simulink model "v2_unittest"  (R2022a)
settings: Solver=VariableStepAuto  StartTime=0.0  StopTime=10.0  RelTol=1e-3
undefined symbols (not defined in the file): sigbuilder_block
libraries: simulink x2
settings Model: Creator=AAMIR  LastModifiedBy=AAMIR

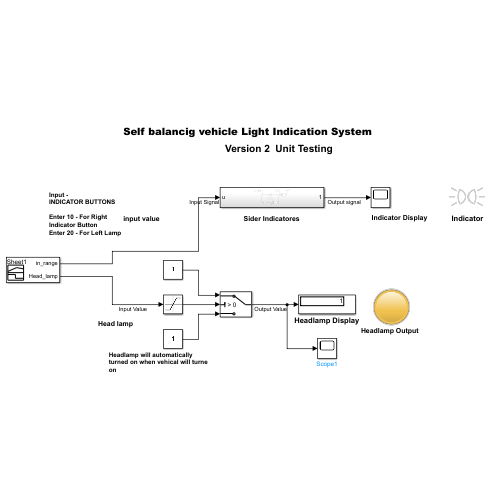
[thumbnail: Simulink's stored preview of the top-level diagram]
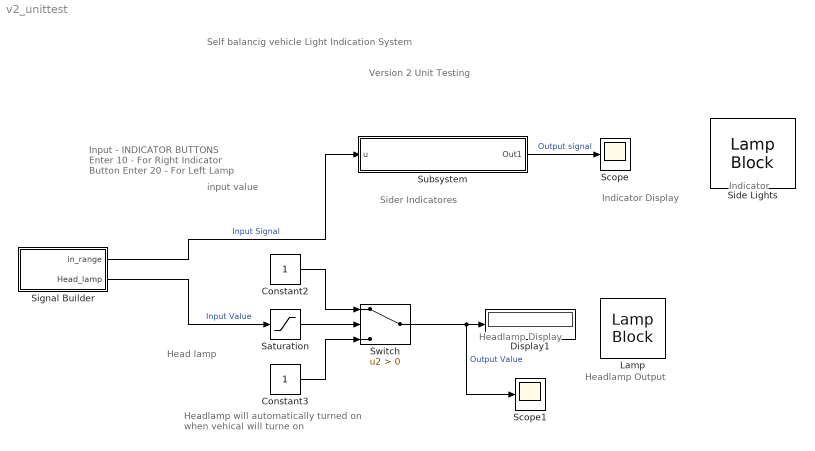
== system v2_unittest ==
  note: input value
  note: Input -
      | INDICATOR BUTTONS
      |
      | Enter 10 - For Right Indicator Button
      | Enter 20 - For Left Lamp
  note: Indicator Display
  note: Head lamp
  note: Self balancig vehicle Light Indication System
  note: Headlamp Output
  note: Indicator
  note: Headlamp will automatically turned on when vehical will turne on
  note: Headlamp Display
  note: Sider Indicatores
  note: Version 2 Unit Testing
  Constant2 : Constant
  Constant3 : Constant
  Display1 : Display
  Lamp : LampBlock  LabelPosition=Hide
  Saturation : Saturate  UpperLimit=1  LowerLimit=0
  Scope : Scope
  Scope1 : Scope
  Side Lights : LampBlock  LabelPosition=Hide  Icon=SideLights
  Signal Builder : Subsystem  Tag=STV Subsys  LoadFcn=sigbuilder_block('load',[437.6 199.2 550.4 400 ]);  StartFcn=sigbuilder_block('start');  StopFcn=sigbuilder_block('stop');  ClipboardFcn=sigbuilder_block('clipboard');  mask(Sigbuilder block){tuvar=[0:10]}
      mask help: Simulink:masks:SigbuilderBlock_MD
      mask init:
      | if ~strcmp(get_param(bdroot(gcbh),'SimulationStatus'),'stopped') tuvar = sigbuilder_block('maskInit'); end
      settings: CopyFcn=sigbuilder_block('copy');  DeleteFcn=sigbuilder_block('delete');  ModelCloseFcn=sigbuilder_block('modelClose');  PreSaveFcn=sigbuilder_block('preSave');  PauseFcn=sigbuilder_block('pause');  ContinueFcn=sigbuilder_block('continue');  NameChangeFcn=sigbuilder_block('namechange');  OpenFcn=sigbuilder_block('open',[437.6 199.2 550.4 400 ]);  CloseFcn=sigbuilder_block('close');
      mask Display: plot(0, 0, 100, 100,[2, 2, 32, 32, 2], [68, 8, 8, 68, 68],[32, 2], [38, 38], [32, 19, 2],[53, 60, 44], [32, 17, 17, 2],[16, 16, 31, 31]);txt = getActiveGroup(gcbh);text(2, 100, txt,'verticalAlignment', 'top');
  Subsystem : Subsystem
  Switch : Switch  Criteria=u2 > Threshold  SaturateOnIntegerOverflow=off  InputSameDT=off
  wires:
  Signal Builder/1(in_range) -> Subsystem/1(u)  "Input Signal"
  Saturation/1 -> Switch/2
  Constant3/1 -> Switch/3
  Constant2/1 -> Switch/1
  Signal Builder/2(Head_lamp) -> Saturation/1  "Input Value"
  Subsystem/1(Out1) -> Scope/1  "Output signal"
  Switch/1 -> Scope1/1, Display1/1  "Output Value"

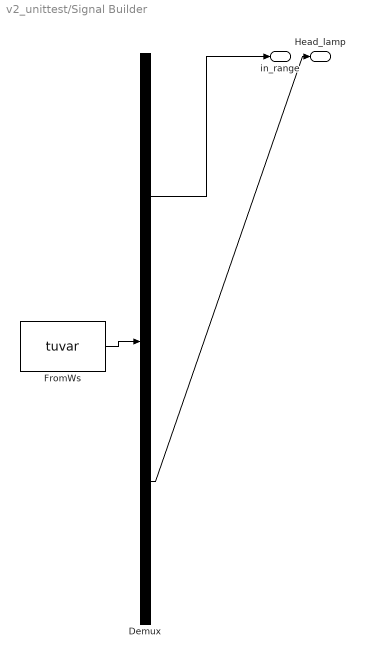
== system v2_unittest/Signal Builder ==
  Demux : Demux  Tag=STV Demux  Outputs=2
      settings: DisplayOption=none
  FromWs : FromWorkspace  Tag=STV FromWs  VariableName=tuvar
      SigBuilderData=|
      | common.afterFinalStr = 'Extrapolate'
      | common.sampleTime = 0
      | dataSet.timeRange = [0.1 1]
      | dataSet.name = 'Sheet1'
      | sbobj.Name = 'Signal Builder'
      | sbobj.Groups.Name = 'Sheet1'
      | sbobj.Groups.Signals(1).Name = 'in_range'
      | sbobj.Groups.Signals(1).XData = [0.1 0.2 0.3 0.4 0.5 0.6 0.7 0.8 0.9 1]
      | sbobj.Groups.Signals(1).YData = [10 20 10 20 10 20 10 20 10 20]
      | sbobj.Groups.Signals(2).Name = 'Head_lamp'
      | sbobj.Groups.Signals(2).XData = [0.1 0.2 0.3 0.4 0.5 0.6 0.7 0.8 0.9 1]
      | sbobj.Groups.Signals(2).YData = [0 1 0 1 0 1 0 1 0 1]
      | sbobj.Groups.TimeRange = [0.1 1]
  in_range : Outport  Tag=STV Outport
  Head_lamp : Outport  Tag=STV Outport  Port=2
  wires:
  Demux/1 -> in_range/1
  FromWs/1 -> Demux/1
  Demux/2 -> Head_lamp/1

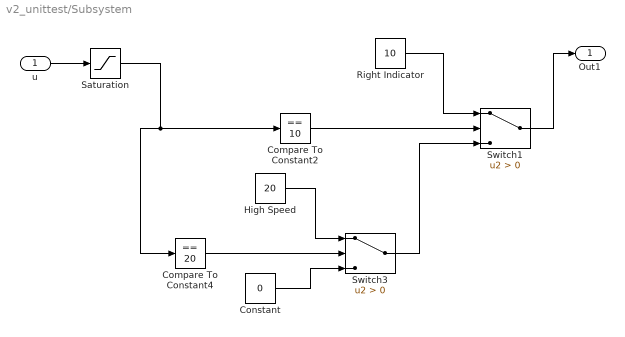
== system v2_unittest/Subsystem ==
  u : Inport
  Compare To Constant2 : simulink/Logic and Bit Operations/Compare To Constant  relop===  const=10  OutDataTypeStr=boolean
  Compare To Constant4 : simulink/Logic and Bit Operations/Compare To Constant  relop===  const=20  OutDataTypeStr=boolean
  Constant : Constant  Value=0
  High Speed : Constant  Value=20
  Right Indicator : Constant  Value=10
  Saturation : Saturate  UpperLimit=20  LowerLimit=0
  Switch1 : Switch  Criteria=u2 > Threshold  SaturateOnIntegerOverflow=off  InputSameDT=off
  Switch3 : Switch  Criteria=u2 > Threshold  SaturateOnIntegerOverflow=off  InputSameDT=off
  Out1 : Outport
  wires:
  Compare To Constant2/1 -> Switch1/2
  u/1 -> Saturation/1
  Compare To Constant4/1 -> Switch3/2
  Switch3/1 -> Switch1/3
  Right Indicator/1 -> Switch1/1
  High Speed/1 -> Switch3/1
  Constant/1 -> Switch3/3
  Switch1/1 -> Out1/1
  Saturation/1 -> Compare To Constant4/1, Compare To Constant2/1
